simulink model "ogranicenje_u_nelin_sim"  (R2020a)
settings: Solver=ode5  StartTime=0.0  StopTime=tfin  FixedStep=1e-4  RelTol=1e-3
values from neighbouring files (symbols this model uses):
  F = Fe    [ogranicenje_u_nelin_sim_matlab.m]
  F_step = 0.002*Fe    [ogranicenje_u_nelin_sim_matlab.m]
  K1 = 0.03    [ogranicenje_u_nelin_sim_matlab.m]
  K2 = 0.5    [ogranicenje_u_nelin_sim_matlab.m]
  mi_max = 1    [ogranicenje_u_nelin_sim_matlab.m]
  SF = 10    [ogranicenje_u_nelin_sim_matlab.m]
  tF_step1 = 2    [ogranicenje_u_nelin_sim_matlab.m]
  tF_step2 = 20    [ogranicenje_u_nelin_sim_matlab.m]
  V = 4    [ogranicenje_u_nelin_sim_matlab.m]
  x10 = Xe    [ogranicenje_u_nelin_sim_matlab.m]
  x20 = Se    [ogranicenje_u_nelin_sim_matlab.m]
  Y = 0.5    [ogranicenje_u_nelin_sim_matlab.m]
undefined symbols (not defined in the file or in its folder): magnitude, std_noise
settings Model: Creator=anaMceranic  LastModifiedBy=anaMceranic
settings DataIOCC: ReturnWorkspaceOutputs=off

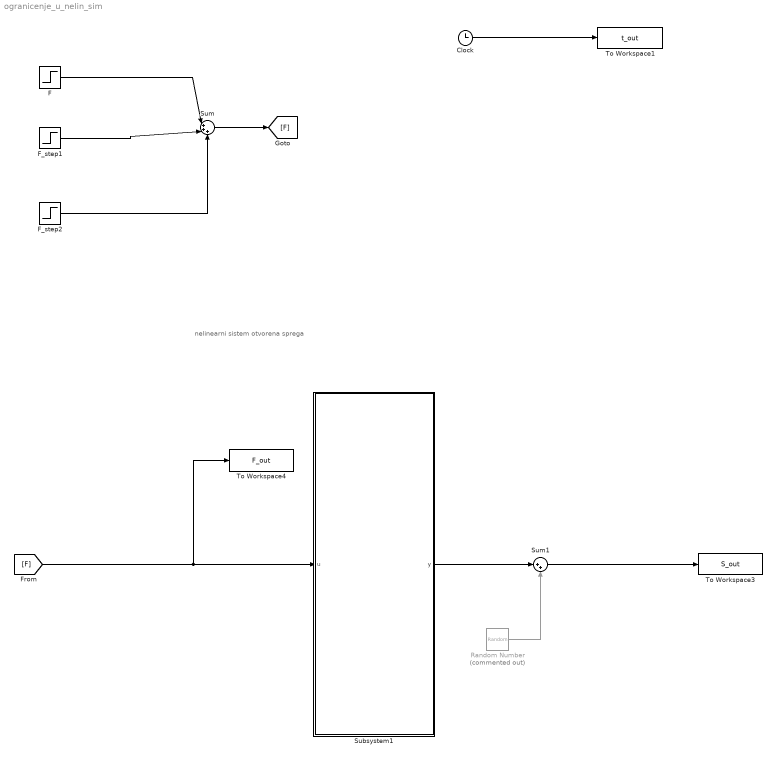
== system ogranicenje_u_nelin_sim ==
  note: nelinearni sistem otvorena sprega
  Clock : Clock
  F : Step  Time=0  After=F  SampleTime=0
  F_step1 : Step  Time=tF_step1  After=F_step  SampleTime=0
  F_step2 : Step  Time=tF_step2  After=-F_step  SampleTime=0
  Random Number : RandomNumber  Commented=on  Variance=std_noise  SampleTime=0.1
  Subsystem1 : Subsystem
  Sum : Sum  Inputs=|+++
  Sum1 : Sum  Inputs=|++
  To Workspace1 : ToWorkspace  VariableName=t_out  SampleTime=-1
  To Workspace3 : ToWorkspace  VariableName=S_out  SampleTime=-1
  To Workspace4 : ToWorkspace  VariableName=F_out  SampleTime=-1
  wires:
  Clock/1 -> To Workspace1/1
  F/1 -> Sum/1
  F_step1/1 -> Sum/2
  F_step2/1 -> Sum/3
  Sum/1 -> [F]
  Subsystem1/1(y) -> Sum1/1
  Random Number/1 -> Sum1/2
  [F] -> To Workspace4/1, Subsystem1/1(u)
  Sum1/1 -> To Workspace3/1

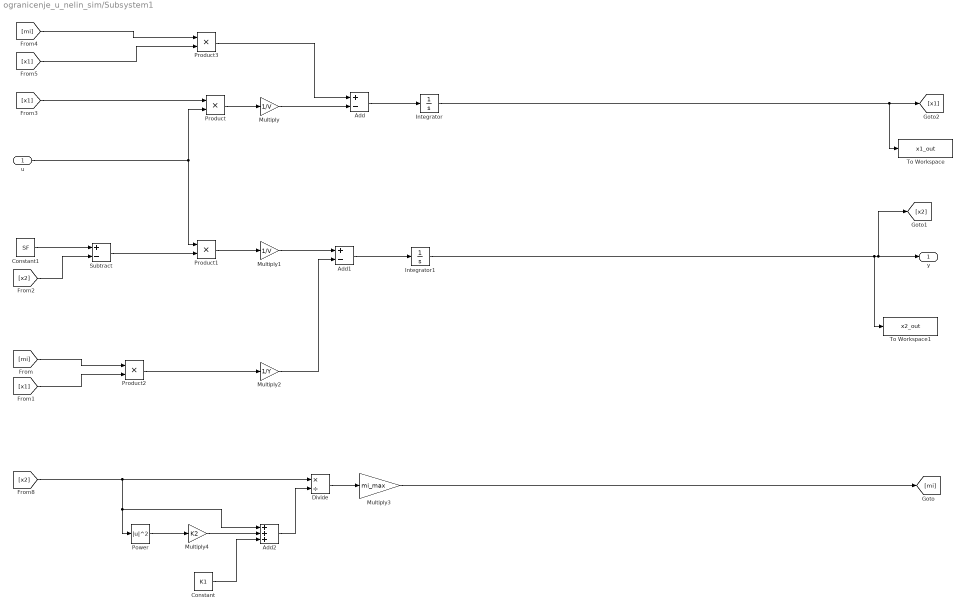
== system ogranicenje_u_nelin_sim/Subsystem1 ==
  u : Inport
  Add : Sum  Inputs=+-
  Add1 : Sum  Inputs=+-
  Add2 : Sum  Inputs=+++
  Constant : Constant  Value=K1
  Constant1 : Constant  Value=SF
  Divide : Product  Inputs=*/
  Integrator : Integrator  InitialCondition=x10
  Integrator1 : Integrator  InitialCondition=x20
  Multiply : Gain  Gain=1/V
  Multiply1 : Gain  Gain=1/V
  Multiply2 : Gain  Gain=1/Y
  Multiply3 : Gain  Gain=mi_max
  Multiply4 : Gain  Gain=K2
  Power : Math  Operator=magnitude^2  SaturateOnIntegerOverflow=on
  Product{,1..3} (4 alike) : Product
  Subtract : Sum  Inputs=+-
  To Workspace : ToWorkspace  VariableName=x1_out  SampleTime=-1
  To Workspace1 : ToWorkspace  VariableName=x2_out  SampleTime=-1
  y : Outport
  wires:
  [x1] -> Product2/2
  Product2/1 -> Multiply2/1
  Multiply/1 -> Add/2
  Add2/1 -> Divide/2
  Constant/1 -> Add2/3
  [x1] -> Product3/2
  Multiply4/1 -> Add2/2
  [mi] -> Product2/1
  Multiply3/1 -> [mi]
  Power/1 -> Multiply4/1
  Constant1/1 -> Subtract/1
  [x2] -> Subtract/2
  Add1/1 -> Integrator1/1
  Multiply2/1 -> Add1/2
  Integrator1/1 -> [x2], y/1, To Workspace1/1
  Divide/1 -> Multiply3/1
  Integrator/1 -> [x1], To Workspace/1
  Product3/1 -> Add/1
  u/1 -> Product1/1, Product/2
  [x1] -> Product/1
  Multiply1/1 -> Add1/1
  Product1/1 -> Multiply1/1
  Subtract/1 -> Product1/2
  [x2] -> Divide/1, Add2/1, Power/1
  Add/1 -> Integrator/1
  Product/1 -> Multiply/1
  [mi] -> Product3/1
